simulink model "Identificacao_Recursiva_NaoLinear"  (R2013b)
settings: Solver=ode45  StartTime=0.0  StopTime=500  RelTol=1e-3
libraries: simulink x1
settings Model: Creator=Eduardo  LastModifiedBy=Eduardo

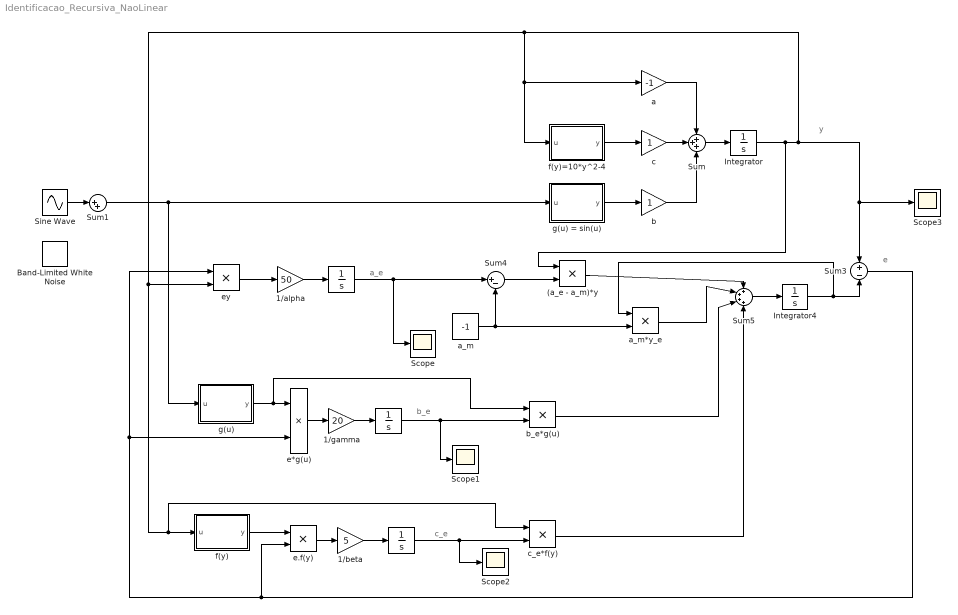
== system Identificacao_Recursiva_NaoLinear ==
  note: c_e
  note: b_e
  note: a_e
  note: e
  note: y
  " " : Integrator
  "  " : Integrator
  "    " : Integrator
  (a_e - a_m)*y : Product
  1/alpha : Gain  Gain=50
  1/beta : Gain  Gain=5
  1/gamma : Gain  Gain=20
  Band-Limited White Noise : simulink/Sources/Band-Limited White Noise  Cov=[0.1]  Ts=0.1  seed=[23341]
  Integrator : Integrator
  Integrator4 : Integrator
  Scope{,1..3} (4 alike) : Scope
      Scope2 settings: SaveName=ScopeData2
      Scope3 settings: SaveName=ScopeData3
  Sine Wave : Sin  SampleTime=0
  Sum : Sum  Inputs=+++
  Sum1 : Sum  Inputs=|++
  Sum3 : Sum  Inputs=+|-
  Sum4 : Sum  Inputs=|+-
  Sum5 : Sum  Inputs=++++
  a : Gain  Gain=-1
  a_m : Constant  Value=-1
  a_m*y_e : Product
  "b " : Gain
  b_e*g(u) : Product
  c : Gain
  "c_e*f(y) " : Product
  e*g(u) : Product
  e.f(y) : Product
  ey : Product
  f(y) : MATLAB Function  TreatAsAtomicUnit=on
  f(y)=10*y^2-4 : MATLAB Function  TreatAsAtomicUnit=on
  g(u) : MATLAB Function  TreatAsAtomicUnit=on
  g(u) = sin(u) : MATLAB Function  TreatAsAtomicUnit=on
  wires:
  a/1 -> Sum/1
  Integrator/1 -> (a_e - a_m)*y/1, Sum3/1, Scope3/1, f(y)=10*y^2-4/1(u), a/1, "c_e*f(y) "/1, f(y)/1(u), ey/2
  f(y)=10*y^2-4/1(y) -> c/1
  c/1 -> Sum/2
  g(u) = sin(u)/1(y) -> "b "/1
  "b "/1 -> Sum/3
  Sum/1 -> Integrator/1
  Sine Wave/1 -> Sum1/1
  Sum1/1 -> g(u)/1(u), g(u) = sin(u)/1(u)
  Sum3/1 -> ey/1, e*g(u)/2, e.f(y)/2
  g(u)/1(y) -> b_e*g(u)/1, e*g(u)/1
  e*g(u)/1 -> 1/gamma/1
  1/gamma/1 -> "  "/1
  ey/1 -> 1/alpha/1
  1/alpha/1 -> " "/1
  f(y)/1(y) -> e.f(y)/1
  e.f(y)/1 -> 1/beta/1
  1/beta/1 -> "    "/1
  a_m/1 -> a_m*y_e/2, Sum4/2
  Sum4/1 -> (a_e - a_m)*y/2
  " "/1 -> Scope/1, Sum4/1
  (a_e - a_m)*y/1 -> Sum5/1
  a_m*y_e/1 -> Sum5/2
  Sum5/1 -> Integrator4/1
  Integrator4/1 -> a_m*y_e/1, Sum3/2
  "  "/1 -> Scope1/1, b_e*g(u)/2
  b_e*g(u)/1 -> Sum5/3
  "c_e*f(y) "/1 -> Sum5/4
  "    "/1 -> Scope2/1, "c_e*f(y) "/2

== matlab function Identificacao_Recursiva_NaoLinear/g(u) = sin(u) ==
  data: u input; y output
function y = g(u)
%#codegen

y = sin(u);

== matlab function Identificacao_Recursiva_NaoLinear/f(y)=10*y^2-4 ==
  data: u input; y output
function y = f(u)
%#codegen

y = u^2;

== matlab function Identificacao_Recursiva_NaoLinear/f(y) ==
  data: u input; y output
function y = f(u)
%#codegen

y = u^2;

== matlab function Identificacao_Recursiva_NaoLinear/g(u) ==
  data: u input; y output
function y = g(u)
%#codegen

y = sin(u);
